simulink model "trigo_mix_test"  (Simulink 9.0)
settings: Solver=FixedStepAuto  StartTime=0.0  StopTime=10.0  FixedStep=0.1  RelTol=1e-3  EnableMultiTasking=on
settings Model: SuppressorTable=22 serialization::archive 11 0 6 0 0 0 0 0  Creator=arnaud  LastModifiedBy=hbourbou
settings DataIOCC: LimitDataPoints=on  SaveFormat=Structure  SignalLoggingSaveFormat=ModelDataLogs
settings OptimizationCC: ExpressionDepthLimit=2147483647
settings DebuggingCC: SolverPrmCheckMsg=warning  FcnCallInpInsideContextMsg=warning  StateNameClashWarn=warning  StrictBusMsg=Warning
settings GRTTargetCC: CombineOutputUpdateFcns=off  GRTInterface=on

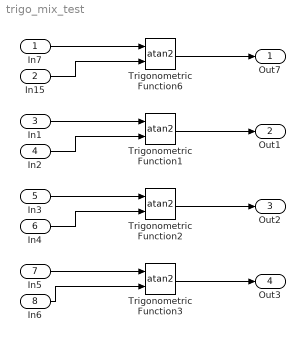
== system trigo_mix_test ==
  In7 : Inport  PortDimensions=1
  In15 : Inport  Port=2  PortDimensions=2
  In1 : Inport  Port=3  PortDimensions=2
  In2 : Inport  Port=4  PortDimensions=1
  In3 : Inport  Port=5  PortDimensions=[2 3]
  In4 : Inport  Port=6  PortDimensions=1
  In5 : Inport  Port=7  PortDimensions=1
  In6 : Inport  Port=8  PortDimensions=[2 3]
  Trigonometric Function{1..3,6} (4 alike) : Trigonometry  Operator=atan2
  Out7 : Outport
  Out1 : Outport  Port=2
  Out2 : Outport  Port=3
  Out3 : Outport  Port=4
  wires:
  In7/1 -> Trigonometric Function6/1
  Trigonometric Function6/1 -> Out7/1
  In15/1 -> Trigonometric Function6/2
  In1/1 -> Trigonometric Function1/1
  Trigonometric Function1/1 -> Out1/1
  In2/1 -> Trigonometric Function1/2
  In3/1 -> Trigonometric Function2/1
  Trigonometric Function2/1 -> Out2/1
  In4/1 -> Trigonometric Function2/2
  In5/1 -> Trigonometric Function3/1
  Trigonometric Function3/1 -> Out3/1
  In6/1 -> Trigonometric Function3/2
